simulink model "PILEncoder"  (R2021a)
settings: Solver=FixedStepAuto  StartTime=0.0  StopTime=41.24  FixedStep=0.001  RelTol=1e-3  EnableMultiTasking=on
values from neighbouring files (symbols this model uses):
  den_lpf_d = den_lpf20    [Mainframe_init.m]    (also in load_autopilot.m)
  Emulated_FCC_IO_Delay = 7    [Mainframe_init.m]
  Enable_Gyros = 0    [Mainframe_init.m]
  Enable_INS = 0    [Mainframe_init.m]
  num_lpf_d = num_lpf20    [Mainframe_init.m]    (also in load_autopilot.m)
undefined symbols (not defined in the file or in its folder): act_dmp, act_omega, Actuator, Aerodynamics, aMode, Autopilot, AUX, c_b_WGS, c_be, c_flat, c_grav, c_h_geop0, c_h_geope, c_pa0, c_pe, c_r0, c_rot, c_rsma, c_Tmp0, d_siB_0, d_siB_max, d_siB_min, dd_siB_max, dd_siB_min, dev, DiscIntNeverNeededParam, e_pa, e_Tmp, Earth, fin_maxrate, flag_I_act_switch, flag_I_aero_switch, flag_I_flat, flag_I_gravity_switch, flag_I_rot, Flight_Logic, hcr, HIL_Data, JMMM_0, JMMM_e, JSPB_e, lat_0, lon_0, Main, Mass_Props, mB_0, mM_0, mM_e, pBII_0, pMPB, pNPB, propellant_kg, prp_FBPB, prp_mdot, prp_T, pSPB, pwm_output0, pwm_output1, qEG_0, qIB_0 ... (+30)
libraries: simulink x42, simulink_extras x24, aerolibcommonsys x4, px4lib x2, custom_blocks x1, dspstat3 x1, pil_lib x1, aerolibtransform2 x1, dspnetwork x1, aerolibnav x1
(part 4 of 16)

== system PILEncoder/Non-linear Flight Dynamic Model/Subsystem1/Extract States/quaternion_to_euler_angles1 ==
  note: Um numerische Probleme zu
      | vermeiden, wird hier eine Saturiierung
      | benutzt.
  note: Outputs [size]:
      |
      | roll angle [1]
      | pitch angle [1]
      | yaw angle [1]
  note: Inputs [size]:
      |
      | quaternion [4]
  q : Inport  PortDimensions=4
  Add : Sum
  Add1 : Sum  Inputs=+--
  Add2 : Sum  Inputs=+-
  Add3 : Sum
  Add4 : Sum  Inputs=+--
  Complex to Real-Imag : ComplexToRealImag  Output=Real
  Constant : Constant  Value=0.5
  Constant1 : Constant  Value=0.5
  Demux : Demux
  Gain : Gain  Gain=2
  Product{,1..9} (10 alike) : Product
  Saturation : Saturate  UpperLimit=1  LowerLimit=-1
      settings: AttributesFormatString=|
      | %<UpperLimit>
      | %<LowerLimit>
  Trigonometric Function : Trigonometry  Operator=atan2
  Trigonometric Function1 : Trigonometry  Operator=asin
  Trigonometric Function2 : Trigonometry  Operator=atan2
  Vector Concatenate : Concatenate  NumInputs=3
  eulx : Outport  VectorParamsAs1DForOutWhenUnconnected=off
  wires:
  Vector Concatenate/1 -> Complex to Real-Imag/1
  Complex to Real-Imag/1 -> eulx/1
  Trigonometric Function2/1 -> Vector Concatenate/3
  Trigonometric Function1/1 -> Vector Concatenate/2
  Trigonometric Function/1 -> Vector Concatenate/1
  Add/1 -> Trigonometric Function/1
  Product1/1 -> Add/2
  Product/1 -> Add/1
  Product3/1 -> Add1/3
  Product2/1 -> Add1/2
  Product5/1 -> Add2/2
  Product4/1 -> Add2/1
  Product7/1 -> Add3/2
  Product6/1 -> Add3/1
  Add3/1 -> Trigonometric Function2/1
  Add4/1 -> Trigonometric Function2/2
  Add2/1 -> Gain/1
  Add1/1 -> Trigonometric Function/2
  q/1 -> Demux/1
  Demux/4 -> Product7/2, Product4/2, Product/2  "4"
  Demux/1 -> Product2/2, Product2/1, Product/1, Product6/1, Product5/1  "1"
  Demux/2 -> Product4/1, Product3/2, Product3/1, Product1/1, Product8/2, Product8/1, Product6/2  "2"
  Constant/1 -> Add1/1
  Product9/1 -> Add4/3
  Product8/1 -> Add4/2
  Constant1/1 -> Add4/1
  Demux/3 -> Product9/2, Product9/1, Product7/1, Product1/2, Product5/2  "3"
  Gain/1 -> Saturation/1
  Saturation/1 -> Trigonometric Function1/1

== system PILEncoder/Non-linear Flight Dynamic Model/Subsystem1/Fin Deflections/Degrees to Radians ==
  Degrees in : Inport
  Gain1 : Gain  Gain=pi/180  SaturateOnIntegerOverflow=on  OutDataTypeStr=Inherit: Same as input  ParamDataTypeStr=Inherit: Same as input
  Radians out : Outport  InitialOutput=0  VectorParamsAs1DForOutWhenUnconnected=off
  wires:
  Gain1/1 -> Radians out/1
  Degrees in/1 -> Gain1/1

== system PILEncoder/Non-linear Flight Dynamic Model/Subsystem1/Fin Deflections/Degrees to Radians1 ==
  Degrees in : Inport
  Gain1 : Gain  Gain=pi/180  SaturateOnIntegerOverflow=on  OutDataTypeStr=Inherit: Same as input  ParamDataTypeStr=Inherit: Same as input
  Radians out : Outport  InitialOutput=0  VectorParamsAs1DForOutWhenUnconnected=off
  wires:
  Gain1/1 -> Radians out/1
  Degrees in/1 -> Gain1/1

== system PILEncoder/Non-linear Flight Dynamic Model/Subsystem1/Fin Deflections/Degrees to Radians2 ==
  Degrees in : Inport
  Gain1 : Gain  Gain=pi/180  SaturateOnIntegerOverflow=on  OutDataTypeStr=Inherit: Same as input  ParamDataTypeStr=Inherit: Same as input
  Radians out : Outport  InitialOutput=0  VectorParamsAs1DForOutWhenUnconnected=off
  wires:
  Gain1/1 -> Radians out/1
  Degrees in/1 -> Gain1/1

== system PILEncoder/Non-linear Flight Dynamic Model/Subsystem1/Fin Deflections/control_allocation ==
  fin_cmd : Inport
  Constant7 : Constant  Value=Tr4r3
  Product : Product  Multiplication=Matrix(*)
  siB_cmd : Outport  VectorParamsAs1DForOutWhenUnconnected=off
  wires:
  Product/1 -> siB_cmd/1  "siB_cmd"
  fin_cmd/1 -> Product/2
  Constant7/1 -> Product/1

== system PILEncoder/Non-linear Flight Dynamic Model/Subsystem1/GRM_Airframe/aerodynamics ==
  str_flow : Inport
  fin : Inport  Port=2
  wab : Inport  Port=3
  env_glbl : Inport  Port=4
  Bus Selector : BusSelector  OutputSignals=qdynB,MaB,alB,beB,hBE,wBIB_star
  Bus Selector1 : BusSelector  OutputSignals=afinB
  Bus Selector2 : BusSelector  OutputSignals=pBPB
  aerodynamic_via_lookup : Subsystem
  logic_base_drag : Subsystem
  aero : Outport  VectorParamsAs1DForOutWhenUnconnected=off
  wires:
  str_flow/1 -> Bus Selector/1
  wab/1 -> Bus Selector2/1
  fin/1 -> Bus Selector1/1
  Bus Selector2/1 -> aerodynamic_via_lookup/1(pBPB)  "<pBPB>"
  Bus Selector/1 -> aerodynamic_via_lookup/2(qdynB)  "<qdynB>"
  Bus Selector/2 -> aerodynamic_via_lookup/3(MaB)  "<MaB>"
  Bus Selector/3 -> aerodynamic_via_lookup/4(alB)  "<alB>"
  Bus Selector/4 -> aerodynamic_via_lookup/5(beB)  "<beB>"
  Bus Selector/5 -> aerodynamic_via_lookup/6(hBE)  "<hBE>"
  Bus Selector1/1 -> aerodynamic_via_lookup/8(afinB)  "<afinB>"
  Bus Selector/6 -> aerodynamic_via_lookup/7(wBIB_star)  "<wBIB_star>"
  aerodynamic_via_lookup/1(aero_bus) -> aero/1
  env_glbl/1 -> logic_base_drag/1(env_glbl)
  logic_base_drag/1(flag_base_drag) -> aerodynamic_via_lookup/9(flag_I_prp)

== system PILEncoder/Non-linear Flight Dynamic Model/Subsystem1/GRM_Airframe/environment ==
  flight_dyn : Inport
  env_glbl : Inport  Port=2
  Bus Creator1 : BusCreator  Inputs=2
  Bus Creator2 : BusCreator  Inputs=2
  Bus Selector : BusSelector  OutputSignals=lon,lat,hBE
  Bus Selector1 : BusSelector  OutputSignals=atm_dyn_bus
  Saturation : Saturate  UpperLimit=inf  LowerLimit=eps
      settings: AttributesFormatString=|
      | %<UpperLimit>
      | %<LowerLimit>
  WGS84_Gravitation : Subsystem  mask{flg_omega_enabled=on}
      mask prompts: flg_omega_enabled "Zentripetalbeschleunigung mitberechnen"
      mask help:
      | Dieser Block berechnet die Gravitation für das idealisierte WGS84
      | Ellipsoid. Die Berechnung ist hierbei nach dem Technical Report
      | "Department of Defense World Geodetic System 1984", NIMA TR8350.2,
      | Third Edition, Amendment 1 vom 3 Januar 2000 implementiert.
      | Das Modell ist gültig für alle Höhen über dem WGS84 Referenzellipsoid, und
      | ist somit der reinen Taylorexpansion des Somigliana Modells überlegen
      | (siehe Kapitel 4.3 des WGS84 reports).
      |
      | ---------------------------------------------------------------------------
      | Longitude [rad]: Nach WGS84 definierte Geodätische Länge.  (lambda)
      | Lattitude [rad]: Nach WGS84 definierte Geodätische Breite. (phi)
      | Height [m]: Höhe über dem WGS84 Referenzellipsoid.
      mask init:
      | [ c_rsma, c_b_WGS, c_grav, c_rot] = init_WGS84_Gravitationsmodell();
  atmosphere_static_ISO_2533 : Subsystem
  convert_to_local_frame : Subsystem
  env : Outport  VectorParamsAs1DForOutWhenUnconnected=off
  wires:
  convert_to_local_frame/1(gBG) -> Bus Creator2/1
  flight_dyn/1 -> Bus Selector/1
  WGS84_Gravitation/1(gE) -> convert_to_local_frame/1(gE)
  Bus Selector/1 -> WGS84_Gravitation/1(lon)  "<lon>"
  Bus Selector/3 -> atmosphere_static_ISO_2533/1(hBE), Saturation/1  "<hBE>"
  Bus Creator2/1 -> env/1  "env_bus"
  Bus Selector/2 -> WGS84_Gravitation/2(lat)  "<lat>"
  Bus Creator1/1 -> Bus Creator2/2  "atm_bus"
  Saturation/1 -> WGS84_Gravitation/3(h)
  atmosphere_static_ISO_2533/1(atm_stat) -> Bus Creator1/1  "atm_stat_bus"
  env_glbl/1 -> Bus Selector1/1, atmosphere_static_ISO_2533/2(env_glbl)
  Bus Selector1/1 -> Bus Creator1/2  "<atm_dyn_bus>"

== system PILEncoder/Non-linear Flight Dynamic Model/Subsystem1/GRM_Airframe/fin_actuators ==
  cmd : Inport
  Bus Creator3 : BusCreator  Inputs=7
  Bus Selector : BusSelector  OutputSignals=siB_cmd
  Constant : Constant  Value=flag_I_act_switch
  Constant7 : Constant  Value=tRRR
  Demux : Demux
  Rudder : Subsystem  mask{siB_max=siB_max, siB_min=siB_min, d_siB_max=d_siB_max, d_siB_min=d_siB_min, dd_siB_max=dd_siB_max, dd_siB_min=dd_siB_min, omega=act_omega, dmp=act_dmp, unc_bl=unc_act_bl, unc_scale=unc_act_scale, unc_off=unc_act_off, siB_0=siB_0, d_siB_0=d_siB_0}
      mask prompts: siB_max "Obere Limitierung des Ruderstellwinkels in [rad]"; siB_min "Untere Limitierung des Ruderstellwinkels in [rad]"; d_siB_max "Obere Limitierung der Ruderstellwinkelgeschwindigkeit in [rad/s]"; d_siB_min "Untere Limitierung der Ruderstellwinkelgeschwindigkeit in [rad/s]"; dd_siB_max "Obere Limitierung der Ruderstellwinkelbeschleunigung in [rad/s^2]"; dd_siB_min "Untere Limitierung der Ruderstellwinkelbeschleunigung in [rad/s^2]"; omega "Eckfrequenz in [Hz]"; dmp "Dämpfung in [kg/s]"; unc_bl "Rückschlag des Aktuators (Backlash) in [rad]"; unc_scale "Skalenfehler in [-]"; unc_off "Versatz (Offset) in [rad]"; siB_0 "Startwert Ruderwinkel in [rad]"; d_siB_0 "Startwert Ruderwinkelgeschwindigkeiten in [rad/s]"
      mask DialogControl ParameterGroupVar Prompt: Limitierungen
      mask DialogControl Container3 Prompt: Dynamik
      mask DialogControl Container4 Prompt: Aktuatorfehler
      mask DialogControl Container5 Prompt: Startwerte
  Rudder1 : Subsystem  mask{siB_max=siB_max, siB_min=siB_min, d_siB_max=d_siB_max, d_siB_min=d_siB_min, dd_siB_max=dd_siB_max, dd_siB_min=dd_siB_min, omega=act_omega, dmp=act_dmp, unc_bl=unc_act_bl, unc_scale=unc_act_scale, unc_off=unc_act_off, siB_0=siB_0, d_siB_0=d_siB_0}
      mask prompts: siB_max "Obere Limitierung des Ruderstellwinkels in [rad]"; siB_min "Untere Limitierung des Ruderstellwinkels in [rad]"; d_siB_max "Obere Limitierung der Ruderstellwinkelgeschwindigkeit in [rad/s]"; d_siB_min "Untere Limitierung der Ruderstellwinkelgeschwindigkeit in [rad/s]"; dd_siB_max "Obere Limitierung der Ruderstellwinkelbeschleunigung in [rad/s^2]"; dd_siB_min "Untere Limitierung der Ruderstellwinkelbeschleunigung in [rad/s^2]"; omega "Eckfrequenz in [Hz]"; dmp "Dämpfung in [kg/s]"; unc_bl "Rückschlag des Aktuators (Backlash) in [rad]"; unc_scale "Skalenfehler in [-]"; unc_off "Versatz (Offset) in [rad]"; siB_0 "Startwert Ruderwinkel in [rad]"; d_siB_0 "Startwert Ruderwinkelgeschwindigkeiten in [rad/s]"
      mask DialogControl ParameterGroupVar Prompt: Limitierungen
      mask DialogControl Container3 Prompt: Dynamik
      mask DialogControl Container4 Prompt: Aktuatorfehler
      mask DialogControl Container5 Prompt: Startwerte
  Rudder2 : Subsystem  mask{siB_max=siB_max, siB_min=siB_min, d_siB_max=d_siB_max, d_siB_min=d_siB_min, dd_siB_max=dd_siB_max, dd_siB_min=dd_siB_min, omega=act_omega, dmp=act_dmp, unc_bl=unc_act_bl, unc_scale=unc_act_scale, unc_off=unc_act_off, siB_0=siB_0, d_siB_0=d_siB_0}
      mask prompts: siB_max "Obere Limitierung des Ruderstellwinkels in [rad]"; siB_min "Untere Limitierung des Ruderstellwinkels in [rad]"; d_siB_max "Obere Limitierung der Ruderstellwinkelgeschwindigkeit in [rad/s]"; d_siB_min "Untere Limitierung der Ruderstellwinkelgeschwindigkeit in [rad/s]"; dd_siB_max "Obere Limitierung der Ruderstellwinkelbeschleunigung in [rad/s^2]"; dd_siB_min "Untere Limitierung der Ruderstellwinkelbeschleunigung in [rad/s^2]"; omega "Eckfrequenz in [Hz]"; dmp "Dämpfung in [kg/s]"; unc_bl "Rückschlag des Aktuators (Backlash) in [rad]"; unc_scale "Skalenfehler in [-]"; unc_off "Versatz (Offset) in [rad]"; siB_0 "Startwert Ruderwinkel in [rad]"; d_siB_0 "Startwert Ruderwinkelgeschwindigkeiten in [rad/s]"
      mask DialogControl ParameterGroupVar Prompt: Limitierungen
      mask DialogControl Container3 Prompt: Dynamik
      mask DialogControl Container4 Prompt: Aktuatorfehler
      mask DialogControl Container5 Prompt: Startwerte
  Rudder3 : Subsystem  mask{siB_max=siB_max, siB_min=siB_min, d_siB_max=d_siB_max, d_siB_min=d_siB_min, dd_siB_max=dd_siB_max, dd_siB_min=dd_siB_min, omega=act_omega, dmp=act_dmp, unc_bl=unc_act_bl, unc_scale=unc_act_scale, unc_off=unc_act_off, siB_0=siB_0, d_siB_0=d_siB_0}
      mask prompts: siB_max "Obere Limitierung des Ruderstellwinkels in [rad]"; siB_min "Untere Limitierung des Ruderstellwinkels in [rad]"; d_siB_max "Obere Limitierung der Ruderstellwinkelgeschwindigkeit in [rad/s]"; d_siB_min "Untere Limitierung der Ruderstellwinkelgeschwindigkeit in [rad/s]"; dd_siB_max "Obere Limitierung der Ruderstellwinkelbeschleunigung in [rad/s^2]"; dd_siB_min "Untere Limitierung der Ruderstellwinkelbeschleunigung in [rad/s^2]"; omega "Eckfrequenz in [Hz]"; dmp "Dämpfung in [kg/s]"; unc_bl "Rückschlag des Aktuators (Backlash) in [rad]"; unc_scale "Skalenfehler in [-]"; unc_off "Versatz (Offset) in [rad]"; siB_0 "Startwert Ruderwinkel in [rad]"; d_siB_0 "Startwert Ruderwinkelgeschwindigkeiten in [rad/s]"
      mask DialogControl ParameterGroupVar Prompt: Limitierungen
      mask DialogControl Container3 Prompt: Dynamik
      mask DialogControl Container4 Prompt: Aktuatorfehler
      mask DialogControl Container5 Prompt: Startwerte
  Switch : Switch  Criteria=u2 > Threshold
  Vector Concatenate1 : Concatenate  NumInputs=4
  Vector Concatenate2 : Concatenate  NumInputs=4
  Vector Concatenate3 : Concatenate  NumInputs=4
  control_allocation : Subsystem
  fin : Outport  VectorParamsAs1DForOutWhenUnconnected=off
  wires:
  [d_siB3] -> Vector Concatenate2/3
  Demux/4 -> Rudder3/1(siB_c)
  Rudder2/2(d_siB) -> [d_siB3]
  Rudder3/1(siB) -> Vector Concatenate1/4
  Rudder1/2(d_siB) -> [d_siB2]
  Rudder2/1(siB) -> Vector Concatenate1/3
  [d_siB4] -> Vector Concatenate2/4
  [d_siB1] -> Vector Concatenate2/1
  Bus Selector/1 -> Switch/3, Demux/1  "<siB_cmd>"
  [d_siB2] -> Vector Concatenate2/2
  Constant7/1 -> Rudder1/2(tRRR), Rudder3/2(tRRR), Rudder2/2(tRRR), Rudder/2(tRRR)
  [dd_siB2] -> Vector Concatenate3/2
  Demux/3 -> Rudder2/1(siB_c)
  Rudder3/2(d_siB) -> [d_siB4]
  Demux/1 -> Rudder/1(siB_c)
  [dd_siB4] -> Vector Concatenate3/4
  [dd_siB3] -> Vector Concatenate3/3
  cmd/1 -> Bus Selector/1
  [dd_siB1] -> Vector Concatenate3/1
  Rudder1/1(siB) -> Vector Concatenate1/2
  Rudder1/3(dd_siB) -> [dd_siB2]
  Rudder3/3(dd_siB) -> [dd_siB4]
  Rudder/2(d_siB) -> [d_siB1]
  Rudder2/3(dd_siB) -> [dd_siB3]
  Demux/2 -> Rudder1/1(siB_c)
  Rudder/3(dd_siB) -> [dd_siB1]
  Rudder/1(siB) -> Vector Concatenate1/1
  Bus Creator3/1 -> fin/1  "fin_bus"
  Switch/1 -> Bus Creator3/1, control_allocation/1(siB)  "siB"
  Vector Concatenate2/1 -> control_allocation/2(d_siB), Bus Creator3/7  "d_siB"
  Vector Concatenate3/1 -> Bus Creator3/6, control_allocation/3(dd_siB)  "dd_siB"
  control_allocation/1(Tr3r4) -> Bus Creator3/2
  control_allocation/2(finB) -> Bus Creator3/3
  control_allocation/3(d_finB) -> Bus Creator3/4
  control_allocation/4(dd_finB) -> Bus Creator3/5
  Vector Concatenate1/1 -> Switch/1  "siB"
  Constant/1 -> Switch/2

== system PILEncoder/Non-linear Flight Dynamic Model/Subsystem1/GRM_Airframe/forces_moments ==
  aero : Inport
  motion_kin : Inport  Port=2
  grav : Inport  Port=3
  prp : Inport  Port=4
  Add : Sum  Inputs=+++
  Add1 : Sum
  Bus Creator : BusCreator  Inputs=2
  Bus Selector : BusSelector  OutputSignals=FBAB,MBAB
  Bus Selector1 : BusSelector  OutputSignals=TGB
  Bus Selector2 : BusSelector  OutputSignals=FBGG
  Bus Selector3 : BusSelector  OutputSignals=FBPB,MBPB
  Math Function : Math  Operator=transpose  SignedPower=on  SaturateOnIntegerOverflow=on
  Product : Product  Multiplication=Matrix(*)
  for_mom_bus : Outport  VectorParamsAs1DForOutWhenUnconnected=off
  wires:
  Bus Selector/1 -> Add/1  "<FBAB>"
  Bus Selector2/1 -> Product/2  "<FBGG>"
  Bus Selector1/1 -> Math Function/1  "<TGB>"
  Math Function/1 -> Product/1  "TBG"
  aero/1 -> Bus Selector/1
  Product/1 -> Add/2  "FBGB"
  prp/1 -> Bus Selector3/1
  motion_kin/1 -> Bus Selector1/1
  Add/1 -> Bus Creator/1  "FBTB"
  grav/1 -> Bus Selector2/1
  Add1/1 -> Bus Creator/2  "MBTB"
  Bus Selector/2 -> Add1/1  "<MBAB>"
  Bus Selector3/1 -> Add/3  "<FBPB>"
  Bus Creator/1 -> for_mom_bus/1  "for_mom_bus"
  Bus Selector3/2 -> Add1/2  "<MBPB>"

== system PILEncoder/Non-linear Flight Dynamic Model/Subsystem1/GRM_Airframe/gravity ==
  env : Inport
  wab : Inport  Port=2
  Bus Creator3 : BusCreator  Inputs=1
  Bus Selector : BusSelector  OutputSignals=gBG,atm_bus.atm_stat_bus.hBE
  Bus Selector1 : BusSelector  OutputSignals=mB
  Product : Product
  launch_rail : Subsystem
  grav : Outport  VectorParamsAs1DForOutWhenUnconnected=off
  wires:
  launch_rail/1(gBG) -> Product/1
  Bus Selector/2 -> launch_rail/2(hBE)  "<hBE>"
  Bus Selector/1 -> launch_rail/1(gBG_c)  "<gBG>"
  Product/1 -> Bus Creator3/1  "FBGG"
  Bus Creator3/1 -> grav/1  "grav_bus"
  wab/1 -> Bus Selector1/1
  Bus Selector1/1 -> Product/2  "<mB>"
  env/1 -> Bus Selector/1

== system PILEncoder/Non-linear Flight Dynamic Model/Subsystem1/GRM_Airframe/input ==
  siB_cmd : Inport
  Bus Creator2 : BusCreator  Inputs=1
  cmd_bus : Outport  VectorParamsAs1DForOutWhenUnconnected=off
  wires:
  siB_cmd/1 -> Bus Creator2/1
  Bus Creator2/1 -> cmd_bus/1  "cmd_bus"

== system PILEncoder/Non-linear Flight Dynamic Model/Subsystem1/GRM_Airframe/motion_kinematics ==
  flight_dyn : Inport
  Bus Creator : BusCreator  Inputs=7
  Bus Selector : BusSelector  OutputSignals=lat,lon,qIB
  calc_motion_kinematics : Subsystem
  motion_kin : Outport  VectorParamsAs1DForOutWhenUnconnected=off
  wires:
  flight_dyn/1 -> Bus Selector/1
  Bus Creator/1 -> motion_kin/1  "motion_kin_bus"
  Bus Selector/1 -> calc_motion_kinematics/1(lat)  "<lat>"
  Bus Selector/2 -> calc_motion_kinematics/2(lon)  "<lon>"
  Bus Selector/3 -> calc_motion_kinematics/3(qIB)  "<qIB>"
  calc_motion_kinematics/1(wIEE) -> Bus Creator/1
  calc_motion_kinematics/2(TIE) -> Bus Creator/2
  calc_motion_kinematics/3(TEB) -> Bus Creator/3
  calc_motion_kinematics/4(TGB) -> Bus Creator/4
  calc_motion_kinematics/5(TEG) -> Bus Creator/5
  calc_motion_kinematics/6(wEGG) -> Bus Creator/6
  calc_motion_kinematics/7(TIB) -> Bus Creator/7

== system PILEncoder/Non-linear Flight Dynamic Model/Subsystem1/GRM_Airframe/propulsion ==
  env_glbl : Inport
  wab : Inport  Port=2
  Bus Creator1 : BusCreator  Inputs=2
  prp_look_up : Subsystem
  prp_uncertainty : Subsystem
  prp : Outport  VectorParamsAs1DForOutWhenUnconnected=off
  wires:
  Bus Creator1/1 -> prp/1  "prp_bus"
  prp_look_up/1(FBPM) -> prp_uncertainty/1(FBPM)
  env_glbl/1 -> prp_look_up/1(env_glbl_bus)
  prp_uncertainty/2(MBPB) -> Bus Creator1/2
  prp_uncertainty/1(FBPB) -> Bus Creator1/1
  wab/1 -> prp_uncertainty/2(wab)

== system PILEncoder/Non-linear Flight Dynamic Model/Subsystem1/GRM_Airframe/rb_eom ==
  mot_kin : Inport
  for_mom : Inport  Port=2
  wab : Inport  Port=3
  Bus Creator : BusCreator  Inputs=16
  calc_bus_flight_dyn_bus_entries : Subsystem
  eom_6dof : Subsystem
  flight_dyn : Outport  VectorParamsAs1DForOutWhenUnconnected=off
  wires:
  mot_kin/1 -> calc_bus_flight_dyn_bus_entries/1(mot_kin)
  calc_bus_flight_dyn_bus_entries/1(aBIB) -> Bus Creator/1
  calc_bus_flight_dyn_bus_entries/2(lon) -> Bus Creator/2
  calc_bus_flight_dyn_bus_entries/3(lat) -> Bus Creator/3
  calc_bus_flight_dyn_bus_entries/4(hBE) -> Bus Creator/4
  calc_bus_flight_dyn_bus_entries/5(vBII) -> Bus Creator/5
  calc_bus_flight_dyn_bus_entries/6(qIB) -> Bus Creator/6
  calc_bus_flight_dyn_bus_entries/7(wBIB) -> Bus Creator/7
  calc_bus_flight_dyn_bus_entries/8(d_wBIB) -> Bus Creator/8
  calc_bus_flight_dyn_bus_entries/9(d_vBII) -> Bus Creator/9
  Bus Creator/1 -> flight_dyn/1  "flight_dyn_bus"
  for_mom/1 -> eom_6dof/1(for_mom)
  wab/1 -> eom_6dof/2(wab)
  eom_6dof/1(eom) -> calc_bus_flight_dyn_bus_entries/2(eom)
  calc_bus_flight_dyn_bus_entries/10(pBII) -> Bus Creator/10
  calc_bus_flight_dyn_bus_entries/11(euIB) -> Bus Creator/11
  calc_bus_flight_dyn_bus_entries/12(vBIB) -> Bus Creator/12
  calc_bus_flight_dyn_bus_entries/13(qGB) -> Bus Creator/13
  calc_bus_flight_dyn_bus_entries/14(euGB) -> Bus Creator/14
  calc_bus_flight_dyn_bus_entries/15(euBG) -> Bus Creator/15
  calc_bus_flight_dyn_bus_entries/16(pBLG) -> Bus Creator/16

== system PILEncoder/Non-linear Flight Dynamic Model/Subsystem1/GRM_Airframe/stream_flow ==
  flight_dyn : Inport
  motion_kin : Inport  Port=2
  env : Inport  Port=3
  Bus Selector1 : BusSelector  OutputSignals=atm_bus.atm_stat_bus.rho,atm_bus.atm_stat_bus.sos,atm_bus.atm_stat_bus.hBE
  Bus Selector2 : BusSelector  OutputSignals=vBII,pBII,wBIB
  Bus Selector3 : BusSelector  OutputSignals=TIB,wIEE,TIE
  calc_stream_flow : Subsystem
  str_flow : Outport  VectorParamsAs1DForOutWhenUnconnected=off
  wires:
  motion_kin/1 -> Bus Selector3/1
  flight_dyn/1 -> Bus Selector2/1
  env/1 -> Bus Selector1/1
  Bus Selector3/1 -> calc_stream_flow/1(TIB)  "<TIB>"
  Bus Selector3/2 -> calc_stream_flow/2(wIEE)  "<wIEE>"
  Bus Selector3/3 -> calc_stream_flow/3(TIE)  "<TIE>"
  Bus Selector2/1 -> calc_stream_flow/4(VBII)  "<vBII>"
  Bus Selector2/3 -> calc_stream_flow/6(wBIB)  "<wBIB>"
  Bus Selector1/1 -> calc_stream_flow/7(rho)  "<rho>"
  Bus Selector1/2 -> calc_stream_flow/8(sos)  "<sos>"
  Bus Selector1/3 -> calc_stream_flow/9(hBE)  "<hBE>"
  calc_stream_flow/1(str_flow) -> str_flow/1
  Bus Selector2/2 -> calc_stream_flow/5(pBII)  "<pBII>"

== system PILEncoder/Non-linear Flight Dynamic Model/Subsystem1/GRM_Airframe/weight_and_balance ==
  env_glb : Inport
  Bus Creator1 : BusCreator  Inputs=3
  Bus Selector2 : BusSelector  OutputSignals=T_sim_glbl,T_sim_lnch
  Subtract : Sum  Inputs=+-
  center_of_gravity : Subsystem
  mass : Subsystem
  mass_uncertainty : Subsystem
  moi : Subsystem
  wab : Outport  VectorParamsAs1DForOutWhenUnconnected=off
  wires:
  Bus Selector2/2 -> Subtract/2  "<T_sim_lnch>"
  Bus Selector2/1 -> Subtract/1  "<T_sim_glbl>"
  env_glb/1 -> Bus Selector2/1
  Bus Creator1/1 -> wab/1  "wab_bus"
  center_of_gravity/1(pBPB) -> moi/1(pBPB), Bus Creator1/2
  moi/1(JBBB) -> Bus Creator1/3
  mass/2(mM) -> moi/2(mM), center_of_gravity/2(mM)
  mass_uncertainty/1(mB) -> center_of_gravity/1(mB), Bus Creator1/1
  mass/1(mB_c) -> mass_uncertainty/1(mB_c)
  Subtract/1 -> mass/1(sim_time_launch)

== system PILEncoder/Flight Control Computer/FCC - Real or Emulated/Emulated FCC/P2R5/Emulated Pixhawk ==
  Serial In : Inport
  100 Hz : DiscretePulseGenerator  PulseType=Time based  Period=0.01  PulseWidth=50
  Autopilot : Subsystem
  Convert to Bus : Subsystem
  Convert to Vector : Subsystem
  IMU - Merge : Subsystem
  Inertial Navigation System : Subsystem
  Real Gyro : Subsystem
  Servo Commands : Subsystem
  Terminator : Terminator
  Zero : Constant  Value=0  OutDataTypeStr=Inherit: Inherit via back propagation
  Serial Out : Outport
  flight_mode_enum : Outport  Port=2
  tag scope: Heartbeat=global
  wires:
  [Heartbeat] -> Convert to Vector/2(Heartbeat)
  [INS_Data] -> Convert to Vector/3(INS Data)
  Serial In/1 -> Convert to Bus/1(Input)
  Convert to Vector/1(To HIL) -> Serial Out/1
  Convert to Bus/4(Missile States) -> Inertial Navigation System/2(Missile States)
  Convert to Bus/6(Virtual IMU Data) -> Real Gyro/1(HIL Gyro), IMU - Merge/1(HIL IMU)
  [INS_Data] -> Autopilot/3(INS Data)
  Real Gyro/1(Gyro Data) -> [Real_Gyro_Data]
  [Real_Gyro_Data] -> Convert to Vector/4(Real Gyro Data)
  [IMU_Data] -> Autopilot/2(IMU Data)
  Inertial Navigation System/1(INS Data) -> [INS_Data]
  Convert to Bus/3(Enable INS Flag) -> Inertial Navigation System/1(Enable INS Flag)
  Convert to Bus/5(Real Gyros Flag) -> Terminator/1
  Convert to Bus/2(Ext. Commands) -> [Ext_Cmd]
  Zero/1 -> Convert to Vector/5(Debug Port)
  IMU - Merge/1(IMU Data) -> [IMU_Data], Inertial Navigation System/3(IMU Data)
  Convert to Bus/1(Heartbeat) -> [Heartbeat]
  [Ext_Cmd] -> Autopilot/1(Cmd)
  Autopilot/1(Fin Deflections) -> Convert to Vector/1(Fin Deflections)
  Autopilot/2(flight_mode_enum) -> flight_mode_enum/1
  100 Hz/1 -> Autopilot/Trigger
  Autopilot/3(Fin Cmd) -> Servo Commands/1(Fin Cmd)
  Autopilot/4(Recovery) -> Servo Commands/2(Recovery)

== system PILEncoder/Flight Control Computer/FCC - Real or Emulated/Real FCC/P2R5/__InputSSForSFun__ ==
  Serial In : Inport
  __UniqueOutportName__1__ : Outport
  wires:
  Serial In/1 -> __UniqueOutportName__1__/1

== system PILEncoder/Flight Control Computer/FCC - Real or Emulated/Real FCC/P2R5/__OutputSSForSFun__ ==
  __UniqueInportName__1__ : Inport
  __UniqueInportName__2__ : Inport  Port=2
  Serial Out : Outport
  flight_mode_enum : Outport  Port=2
  wires:
  __UniqueInportName__2__/1 -> flight_mode_enum/1  "flight_mode_enum"
  __UniqueInportName__1__/1 -> Serial Out/1

== system PILEncoder/Flight Control Computer/FCC - Real or Emulated/Real FCC/PixBlock2/Emulated Pixhawk ==
  Serial In : Inport
  Trigger : TriggerPort  VariantControl=Variant  PortDimensions=1
  Autopilot : Subsystem
  Convert to Bus : Subsystem
  Convert to Vector : Subsystem
  Fin Allocation : Subsystem
  IMU - Merge : Subsystem
  Inertial Navigation System : Subsystem
  Real Gyro : Subsystem
  Servo Commands : Subsystem  Commented=on
  Terminator : Terminator
  Zero : Constant  Value=0  OutDataTypeStr=Inherit: Inherit via back propagation
  Serial Out : Outport
  tag scope: Heartbeat=global
  wires:
  [Heartbeat] -> Convert to Vector/2(Heartbeat)
  [INS_Data] -> Convert to Vector/3(INS Data)
  Serial In/1 -> Convert to Bus/1(Input)
  Convert to Vector/1(To HIL) -> Serial Out/1
  Convert to Bus/4(Missile States) -> Inertial Navigation System/2(Missile States)
  Convert to Bus/6(Virtual IMU Data) -> Real Gyro/1(HIL Gyro), IMU - Merge/1(HIL IMU)
  [INS_Data] -> Autopilot/3(INS Data)
  Real Gyro/1(Gyro Data) -> [Real_Gyro_Data]
  Fin Allocation/1(Fin Cmd) -> Servo Commands/1(Fin Cmd), Convert to Vector/1(Fin Deflections)
  Autopilot/1(Attitude_Commands) -> Fin Allocation/1(Attitude Cmd)  "ATT_Cmd"
  [Real_Gyro_Data] -> Convert to Vector/4(Real Gyro Data)
  [IMU_Data] -> Autopilot/2(IMU Data)
  Inertial Navigation System/1(INS Data) -> [INS_Data]
  Convert to Bus/3(Enable INS Flag) -> Inertial Navigation System/1(Enable INS Flag)
  Convert to Bus/5(Real Gyros Flag) -> Terminator/1
  Convert to Bus/2(Ext. Commands) -> [Ext_Cmd]
  Zero/1 -> Convert to Vector/5(Debug Port)
  IMU - Merge/1(IMU Data) -> [IMU_Data], Inertial Navigation System/3(IMU Data)
  Convert to Bus/1(Heartbeat) -> [Heartbeat]
  [Ext_Cmd] -> Autopilot/1(Cmd)

== system PILEncoder/Non-linear Flight Dynamic Model/Environment/atm_dynamic/trafo_around_z_axis/1_rot_mat ==
  wi1 : Inport
  1. Rotation x-Achse : Subsystem
  1. Rotation y-Achse : Subsystem
  1. Rotation z-Achse : Subsystem
  Constant : Constant  Value=rot_1
  Multiport Switch : MultiPortSwitch
  T12 : Outport  VectorParamsAs1DForOutWhenUnconnected=off
  wires:
  Constant/1 -> Multiport Switch/1
  1. Rotation x-Achse/1(1Rot_Matrix_x) -> Multiport Switch/2
  1. Rotation y-Achse/1(1Rot_Matrix_y) -> Multiport Switch/3
  1. Rotation z-Achse/1(1Rot_Matrix_z) -> Multiport Switch/4
  wi1/1 -> 1. Rotation x-Achse/1(alpha1), 1. Rotation z-Achse/1(alpha1), 1. Rotation y-Achse/1(alpha1)
  Multiport Switch/1 -> T12/1  "T12"

== system PILEncoder/Non-linear Flight Dynamic Model/Extract States/Assemble_States_Bus1/Three-axis Inertial Measurement Unit3/Acceleration Conversion ==
  acceleration : Inport  Unit=m/s^2
  Unit Conversion : UnitConversion
  inherit : Outport  VectorParamsAs1DForOutWhenUnconnected=off
  wires:
  acceleration/1 -> Unit Conversion/1
  Unit Conversion/1 -> inherit/1

== system PILEncoder/Non-linear Flight Dynamic Model/Extract States/Assemble_States_Bus1/Three-axis Inertial Measurement Unit3/Three-axis Accelerometer ==
  Ab : Inport  Unit=m/s^2  PortDimensions=3
  p q r : Inport  Port=2  Unit=rad/s
  pdot qdot rdot : Inport  Port=3  Unit=rad/s^2
  CG : Inport  Port=4  Unit=m  PortDimensions=3
  g : Inport  Port=5  Unit=m/s^2
  Disallow CGS : UnitConfiguration  UnitSystemsStr=English,SI,SI (extended)  AllowAllUnitSystems=off
  Dynamics : Subsystem
  Gain : Gain  Gain=[1 -1 1]  SaturateOnIntegerOverflow=on  OutDataTypeStr=Inherit: Same as input  ParamDataTypeStr=Inherit: Same as input
  Measurement bias : Constant  Value=a_bias
  Product : Product  Multiplication=Matrix(*)  SaturateOnIntegerOverflow=on  OutDataTypeStr=Inherit: Same as first input
  Random bias : aerolibcommonsys/Tunable White Noise  pwr=a_pow  Ts=0.1  seed=a_seeds
      settings: SourceProductBaseCode=AE
  Reshape1 : Reshape
  Saturation : Saturate  UpperLimit=a_sath  LowerLimit=a_satl
  Scale factors & Cross-coupling errors : Constant  Value=a_sf_cc
  Sum : Sum  Inputs=+-++  SaturateOnIntegerOverflow=on
  Sum1 : Sum  Inputs=|++  SaturateOnIntegerOverflow=on
  Sum4 : Sum  Inputs=++|  SaturateOnIntegerOverflow=on
  Sum7 : Sum  Inputs=|+-  SaturateOnIntegerOverflow=on
  Zero-Order Hold{,1..4} (5 alike) : Gain  SaturateOnIntegerOverflow=on  OutDataTypeStr=Inherit: Same as input  ParamDataTypeStr=Inherit: Same as input
  w x (w x d) : Subsystem
  wdot x d : Subsystem  mask(CrossProduct){aMode=aMode}
      mask help: shared_aeroblks:sharedaeroblkutil:blockCrossProductDesc
      mask init:
      | if aerosharedtest(gcb)
      |     aerosharedicon('shared');
      | else
      |     sharedautoicon('shared');
      | end
      mask Help: eval('if license(''test'',''Aerospace_Blockset'')aerosharedhelp(''threebythree_cross_product'');elseif license(''test'',''Powertrain_Blockset'')sharedautohelp(''threebythree_cross_product'');end')
      mask Display:
      | text(.5,.5,'Cross\nProduct\nC = AxB', ...
      | 	'HorizontalAlignment','Center',...
      | 	'VerticalAlignment','middle')
  wl_ins : Constant  Value=acc
  Ameas : Outport  Unit=m/s^2  PortDimensions=3  VectorParamsAs1DForOutWhenUnconnected=off
  wires:
  Zero-Order Hold4/1 -> Sum7/1
  Zero-Order Hold3/1 -> wdot x d/1(A)
  Zero-Order Hold/1 -> w x (w x d)/1("p q r ")
  Zero-Order Hold2/1 -> Sum/2
  Zero-Order Hold1/1 -> Sum/1
  g/1 -> Zero-Order Hold2/1
  Gain/1 -> wdot x d/2(B), w x (w x d)/2(distance)
  wl_ins/1 -> Sum7/2
  Sum7/1 -> Gain/1
  Dynamics/1("sp_f ") -> Sum1/1
  Sum4/1 -> Dynamics/1(sp_f)
  Sum1/1 -> Saturation/1
  w x (w x d)/1(w x ( w x d)) -> Sum/3
  Ab/1 -> Zero-Order Hold1/1
  Reshape1/1 -> Sum4/1
  Measurement bias/1 -> Sum4/2
  Product/1 -> Reshape1/1
  CG/1 -> Zero-Order Hold4/1
  pdot qdot rdot/1 -> Zero-Order Hold3/1
  p q r/1 -> Zero-Order Hold/1
  Sum/1 -> Product/2
  wdot x d/1(C) -> Sum/4
  Scale factors & Cross-coupling errors/1 -> Product/1
  Random bias/1 -> Sum1/2
  Saturation/1 -> Ameas/1

== system PILEncoder/Non-linear Flight Dynamic Model/Extract States/Assemble_States_Bus1/Three-axis Inertial Measurement Unit3/Three-axis Gyroscope ==
  p q r : Inport  Unit=rad/s  PortDimensions=3
  G's : Inport  Port=2  Unit=gn  PortDimensions=3
  Disallow CGS : UnitConfiguration  UnitSystemsStr=English,SI,SI (extended)  AllowAllUnitSystems=off
  Dynamics : Subsystem
  Measurement bias : Constant  Value=g_bias
  Product : Product  Multiplication=Matrix(*)  SaturateOnIntegerOverflow=on  OutDataTypeStr=Inherit: Same as first input
  Product1 : Product  SaturateOnIntegerOverflow=on  OutDataTypeStr=Inherit: Same as first input
  Random bias : aerolibcommonsys/Tunable White Noise  pwr=g_pow  Ts=0.1  seed=g_seeds
      settings: SourceProductBaseCode=AE
  Saturation : Saturate  UpperLimit=g_sath  LowerLimit=g_satl
  "Scale factors & Cross-coupling errors " : Constant  Value=g_sf_cc
  Sum1 : Sum  Inputs=|++  SaturateOnIntegerOverflow=on
  Sum4 : Sum  Inputs=+++  SaturateOnIntegerOverflow=on
  Zero-Order Hold : Gain  SaturateOnIntegerOverflow=on  OutDataTypeStr=Inherit: Same as input  ParamDataTypeStr=Inherit: Same as input
  Zero-Order Hold1 : Gain  SaturateOnIntegerOverflow=on  OutDataTypeStr=Inherit: Same as input  ParamDataTypeStr=Inherit: Same as input
  g-sensitive bias : Constant  Value=g_sen
  (p q r)_meas : Outport  Unit=rad/s  PortDimensions=3  VectorParamsAs1DForOutWhenUnconnected=off
  wires:
  Zero-Order Hold1/1 -> Product1/1
  Zero-Order Hold/1 -> Product/2
  Product1/1 -> Sum4/3
  Dynamics/1("p q r ") -> Sum1/1
  G's/1 -> Zero-Order Hold1/1
  Sum1/1 -> Saturation/1
  g-sensitive bias/1 -> Product1/2
  p q r/1 -> Zero-Order Hold/1
  Saturation/1 -> (p q r)_meas/1
  Random bias/1 -> Sum1/2
  "Scale factors & Cross-coupling errors "/1 -> Product/1
  Sum4/1 -> Dynamics/1(p q r)
  Product/1 -> Sum4/1
  Measurement bias/1 -> Sum4/2

== system PILEncoder/Non-linear Flight Dynamic Model/GRM_Airframe/aerodynamics/aerodynamic_via_lookup/calc_aero_coefficients ==
  dela_deg : Inport
  dele_deg : Inport  Port=2
  delr_deg : Inport  Port=3
  pBIB_star_rps : Inport  Port=4
  qBIB_star_rps : Inport  Port=5
  rBIB_star_rps : Inport  Port=6
  alB_deg : Inport  Port=7
  beB_deg : Inport  Port=8
  CLL_TLU : Subsystem
  CLM_TLU : Subsystem
  CLN_TLU : Subsystem
  CX_TLU : Subsystem
  CY_TLU : Subsystem
  CZ_TLU : Subsystem
  alB_deg D{1..5} (5 alike) : InportShadow  Port=7
  beB_deg D{1..5} (5 alike) : InportShadow  Port=8
  dela_deg D{1..6} (6 alike) : InportShadow
  dele_deg D{1..4} (4 alike) : InportShadow  Port=2
  delr_deg D{1..5} (5 alike) : InportShadow  Port=3
  Cx : Outport  VectorParamsAs1DForOutWhenUnconnected=off
  Cy : Outport  Port=2  VectorParamsAs1DForOutWhenUnconnected=off
  Cz : Outport  Port=3  VectorParamsAs1DForOutWhenUnconnected=off
  Cl : Outport  Port=4  VectorParamsAs1DForOutWhenUnconnected=off
  Cm : Outport  Port=5  VectorParamsAs1DForOutWhenUnconnected=off
  Cn : Outport  Port=6  VectorParamsAs1DForOutWhenUnconnected=off
  wires:
  CX_TLU/1(CX) -> Cx/1
  alB_deg/1 -> CX_TLU/1(alpha_deg)
  beB_deg/1 -> CX_TLU/2(beta_deg)
  dele_deg/1 -> CX_TLU/3(dele_deg)
  dela_deg/1 -> CX_TLU/4(dela_deg)
  CY_TLU/1(CY) -> Cy/1
  beB_deg D1/1 -> CY_TLU/2(beta_deg)
  alB_deg D1/1 -> CY_TLU/1(alpha_deg)
  delr_deg/1 -> CX_TLU/5(delr_deg)
  CZ_TLU/1(CZ) -> Cz/1
  CLL_TLU/1(CLL) -> Cl/1
  CLM_TLU/1(CLM) -> Cm/1
  CLN_TLU/1(CLN) -> Cn/1
  pBIB_star_rps/1 -> CLL_TLU/6(p_ND_rps)
  qBIB_star_rps/1 -> CLM_TLU/6(q_ND_rps)
  rBIB_star_rps/1 -> CLN_TLU/6(r_ND_rps)
  alB_deg D2/1 -> CZ_TLU/1(alpha_deg)
  beB_deg D2/1 -> CZ_TLU/2(beta_deg)
  dele_deg D1/1 -> CY_TLU/3(dele_deg)
  dela_deg D1/1 -> CY_TLU/4(dela_deg)
  delr_deg D1/1 -> CY_TLU/5(delr_deg)
  dele_deg D2/1 -> CZ_TLU/3(dele_deg)
  dela_deg D2/1 -> CZ_TLU/4(dela_deg)
  delr_deg D2/1 -> CZ_TLU/5(delr_deg)
  dela_deg D3/1 -> CLN_TLU/3(dele_deg)
  dela_deg D4/1 -> CLN_TLU/4(dela_deg)
  delr_deg D3/1 -> CLN_TLU/5(delr_deg)
  alB_deg D5/1 -> CLN_TLU/1(alpha_deg)
  alB_deg D4/1 -> CLM_TLU/1(alpha_deg)
  alB_deg D3/1 -> CLL_TLU/1(alpha_deg)
  beB_deg D3/1 -> CLL_TLU/2(beta_deg)
  beB_deg D4/1 -> CLM_TLU/2(beta_deg)
  beB_deg D5/1 -> CLN_TLU/2(beta_deg)
  dele_deg D3/1 -> CLL_TLU/3(dele_deg)
  dele_deg D4/1 -> CLM_TLU/3(dele_deg)
  dela_deg D5/1 -> CLL_TLU/4(dela_deg)
  dela_deg D6/1 -> CLM_TLU/4(dela_deg)
  delr_deg D4/1 -> CLL_TLU/5(delr_deg)
  delr_deg D5/1 -> CLM_TLU/5(delr_deg)

== system PILEncoder/Non-linear Flight Dynamic Model/GRM_Airframe/aerodynamics/aerodynamic_via_lookup/calc_aero_for_mom ==
  hBE : Inport
  pBPB : Inport  Port=2
  qdynB : Inport  Port=3
  Cx : Inport  Port=4
  Cy : Inport  Port=5
  Cz : Inport  Port=6
  Cl : Inport  Port=7
  Cm : Inport  Port=8
  Cn : Inport  Port=9
  Add : Sum
  Constant1 : Constant  Value=Aerodynamics.lref
      settings: AttributesFormatString=%<Value>
  Constant2 : Constant  Value=Aerodynamics.sref
      settings: AttributesFormatString=%<Value>
  Product : Product
  Product1 : Product  Inputs=3
  Product2 : Product
  Subtract : Sum  Inputs=+-
  Vector Concatenate1 : Concatenate  NumInputs=3
  Vector Concatenate2 : Concatenate  NumInputs=3
  create_pAPB : Subsystem
  cross_product : Subsystem
      mask help: cross product r3 = r1 x r2
      mask Help:
      | Name:
      | 
      |     cross_product
      | 
      | Description:
      | 
      |     This block implements the cross product r3 = r1 x r2.
      | 
      | Inputs  [size] [data type] [unit]:
      | 
      |     vector 1  [3] [double] [-]
      |     vector 2  [3] [double] [-]
      | 
      | Outputs  [size] [data type] [unit]:
      | 
      |     resulting vector  [3] [double] [-]
      mask Display: disp(' r3 = r1 x r2')
  launch_rail : Subsystem
  launch_rail1 : Subsystem
  FBAB : Outport  VectorParamsAs1DForOutWhenUnconnected=off
  MBAB : Outport  Port=2  VectorParamsAs1DForOutWhenUnconnected=off
  wires:
  Cy/1 -> Vector Concatenate2/2
  Cm/1 -> Vector Concatenate1/2
  Cz/1 -> Vector Concatenate2/3
  Cx/1 -> Vector Concatenate2/1
  Cl/1 -> Vector Concatenate1/1
  Cn/1 -> Vector Concatenate1/3
  qdynB/1 -> Product2/2
  Vector Concatenate1/1 -> Product1/2
  Vector Concatenate2/1 -> Product/1
  pBPB/1 -> Subtract/2
  Product/1 -> launch_rail/2(FBAB_c), cross_product/2(r2)  "FBAB"
  Product1/1 -> Add/2  "MBAB"
  Add/1 -> launch_rail1/2(MBAB_c)  "MBAB"
  Constant1/1 -> Product1/3
  Constant2/1 -> Product2/1
  Product2/1 -> Product1/1, Product/2
  cross_product/1(r1_x_r2) -> Add/1
  hBE/1 -> launch_rail1/1(hBE), launch_rail/1(hBE)
  launch_rail1/1(MBAB) -> MBAB/1
  launch_rail/1(FBAB) -> FBAB/1
  Subtract/1 -> cross_product/1(r1)  "pBAB"
  create_pAPB/1(pAPB) -> Subtract/1

== system PILEncoder/Non-linear Flight Dynamic Model/GRM_Airframe/environment/WGS84_Gravitation/WGS84_2_ECEF ==
  h : Inport
  lon : Inport  Port=2
  lat : Inport  Port=3
  Add1 : Sum  Inputs=+-
  Add2 : Sum
  Add3 : Sum
  Constant : Constant
  Divide : Product  Inputs=***
  Divide1 : Product  Inputs=***
  Divide2 : Product  Inputs=**
  Divide3 : Product  Inputs=**
  Divide4 : Product  Inputs=**
  Mux : Mux  Inputs=3
  Trigonometric Function : Trigonometry
  Trigonometric Function1 : Trigonometry  Operator=cos
  Trigonometric Function2 : Trigonometry
  Trigonometric Function3 : Trigonometry  Operator=cos
  "WGS84 Transformation Parameter " : Subsystem
  pE : Outport  VectorParamsAs1DForOutWhenUnconnected=off
  wires:
  Divide1/1 -> Mux/2  "y_ECEF"
  Add2/1 -> Divide4/1
  Divide/1 -> Mux/1  "x_ECEF"
  lat/1 -> "WGS84 Transformation Parameter "/1(phi), Trigonometric Function3/1, Trigonometric Function2/1
  Divide2/1 -> Add1/2
  Divide3/1 -> Add2/2  "N(1-e^2)"
  Constant/1 -> Add1/1
  Add1/1 -> Divide3/2
  Divide4/1 -> Mux/3  "z_ECEF"
  "WGS84 Transformation Parameter "/1(N) -> Add3/2, Divide3/1
  "WGS84 Transformation Parameter "/2(e) -> Divide2/2, Divide2/1
  h/1 -> Add2/1, Add3/1
  Trigonometric Function1/1 -> Divide/2  "cos(lambda)"
  Trigonometric Function3/1 -> Divide1/3, Divide/3  "cos(phi)"
  Mux/1 -> pE/1  "pE"
  lon/1 -> Trigonometric Function1/1, Trigonometric Function/1
  Add3/1 -> Divide1/1, Divide/1
  Trigonometric Function2/1 -> Divide4/2  "sin(phi)"
  Trigonometric Function/1 -> Divide1/2  "sin(lambda)"

== system PILEncoder/Non-linear Flight Dynamic Model/GRM_Airframe/environment/atmosphere_static_ISO_2533/density ==
  Tmp : Inport
  pa : Inport  Port=2
  Divide : Product  Inputs=/*/
  specific_gas_constant : Constant  Value=sgc
  rho : Outport  VectorParamsAs1DForOutWhenUnconnected=off
  wires:
  Tmp/1 -> Divide/1
  Divide/1 -> rho/1  "rho"
  pa/1 -> Divide/2
  specific_gas_constant/1 -> Divide/3

== system PILEncoder/Non-linear Flight Dynamic Model/GRM_Airframe/environment/atmosphere_static_ISO_2533/geopot_height ==
  hBE : Inport
  Add : Sum
  Divide : Product  Inputs=*/*
  mean_earth_radius : Constant  Value=mean_earth_radius
  h_geop : Outport  VectorParamsAs1DForOutWhenUnconnected=off
  wires:
  mean_earth_radius/1 -> Divide/3, Add/2
  Divide/1 -> h_geop/1  "h_geop"
  hBE/1 -> Add/1, Divide/1
  Add/1 -> Divide/2

== system PILEncoder/Non-linear Flight Dynamic Model/GRM_Airframe/environment/atmosphere_static_ISO_2533/speed_of_sound ==
  Tmp : Inport
  Product : Product  Inputs=3
  Sqrt : Sqrt  SaturateOnIntegerOverflow=on
  heat_capacity_ratio : Constant  Value=hcr
  specific_gas_constant : Constant  Value=sgc
  sos : Outport  VectorParamsAs1DForOutWhenUnconnected=off
  wires:
  Sqrt/1 -> sos/1  "sos"
  Tmp/1 -> Product/3
  Product/1 -> Sqrt/1
  heat_capacity_ratio/1 -> Product/2
  specific_gas_constant/1 -> Product/1

== system PILEncoder/Non-linear Flight Dynamic Model/GRM_Airframe/environment/atmosphere_static_ISO_2533/tmp_and_pressure_ISO_2533 ==
  h_geop : Inport
  e_Tmp : Inport  Port=2
  e_pa : Inport  Port=3
  Subtract1 : Sum
  Subtract2 : Sum
  Tmp_norm_msl : Constant  Value=c_Tmp0
  geopotential_height_ref : Constant  Value=c_h_geop0
  pa_norm_msl : Constant  Value=c_pa0
  static_Temperature : Subsystem
  static_pressure : Subsystem
  Tmp : Outport  VectorParamsAs1DForOutWhenUnconnected=off
  pa : Outport  Port=2  VectorParamsAs1DForOutWhenUnconnected=off
  wires:
  h_geop/1 -> static_pressure/2(h_geop), static_Temperature/2(h_geop)
  Subtract2/1 -> static_pressure/4(pa_ref)  "pa_ref"
  pa_norm_msl/1 -> Subtract2/2
  Subtract1/1 -> static_pressure/3(Tmp_ref), static_Temperature/1(Tmp_ref)  "Tmp_ref"
  static_pressure/1(pa) -> pa/1
  e_pa/1 -> Subtract2/1
  static_Temperature/1(Tmp) -> Tmp/1
  e_Tmp/1 -> Subtract1/1
  geopotential_height_ref/1 -> static_pressure/1(h_geop_ref), static_Temperature/3(h_geop_ref)  "h_geop_ref"
  Tmp_norm_msl/1 -> Subtract1/2

== system PILEncoder/Non-linear Flight Dynamic Model/GRM_Airframe/gravity/launch_rail/initial_altitude ==
  Constant : Constant  Value=pBII_0
  Constant2 : Constant  Value=flag_I_flat
  Demux : Demux  Outputs=3
  Gain : Gain  Gain=-1
  Switch1 : Switch  Criteria=u2 > Threshold
  Terminator{,1..3} (4 alike) : Terminator
  trafo_E_to_geodetic : Subsystem  mask(Transformation der ECEF Position in geodätische Größen){}
      mask help: Dieser Block transformiert die Position im ECEF KOS in die geodätische Länge, Breite und Höhe
      mask init:
      | [c_mue, c_rsma, c_flat] = init_transformations_earth;
      mask Help:
      | Name:
      | 
      |     trafo_E_to_geodetic
      | 
      | Beschreibung:
      | 
      |     Dieser Block transformiert die Position im ECEF KOS in die geodätische
      |     Länge, Breite und Höhe.
      | 
      | Inputs   [size]  [data type] [unit]:
      | 
      |     pBEE    [3] [double] [m]
      | 
      | Outputs  [size]  [data type] [unit]:
      | 
      |     long  [1] [double] [rad]
      |     lat   [1] [double] [rad]
      |     alt   [1] [double] [m]
      | 
      | Parameter
      | 
      |    c_rsma
      |    c_flat
  hBE_0 : Outport  VectorParamsAs1DForOutWhenUnconnected=off
  wires:
  Constant2/1 -> Switch1/2
  trafo_E_to_geodetic/3(alt) -> Switch1/3  "hBE_0"
  Demux/2 -> Terminator3/1
  Demux/3 -> Gain/1
  Gain/1 -> Switch1/1
  Demux/1 -> Terminator2/1
  trafo_E_to_geodetic/2(lat) -> Terminator1/1
  Constant/1 -> Demux/1, trafo_E_to_geodetic/1(pBEE)
  trafo_E_to_geodetic/1(lon) -> Terminator/1
  Switch1/1 -> hBE_0/1  "hBE_0"

== system PILEncoder/Non-linear Flight Dynamic Model/GRM_Airframe/motion_kinematics/calc_motion_kinematics/calc_transformation_matrix ==
  qIE : Inport
  qEG : Inport  Port=2
  qIB : Inport  Port=3
  T12_from_q1 : Subsystem
      mask help: Transforms a quaternion into a Direction Cosine Matrix
      mask Help:
      | Name:
      | 
      |     T12_from_q12
      | 
      | Description:
      | 
      |     This block implements the transformation of a quaternion into the
      |     corresponding direction cosine matrix DCM.
      | 
      | Inputs  [size] [data type] [unit]:
      | 
      |     quaternion q12 [4] [double] [-]
      | 
      | Outputs  [size] [data type] [unit]:
      | 
      |     direction cosine matrix T12  [3x3] [double] [-]
      mask Display:
      | %port_label('input', 1, 'q12')
      | %port_label('output', 1, 'T12')
      | disp('q \rightarrow DCM','texmode','on')
  T12_from_q12 : Subsystem
      mask help: Transforms a quaternion into a Direction Cosine Matrix
      mask Help:
      | Name:
      | 
      |     T12_from_q12
      | 
      | Description:
      | 
      |     This block implements the transformation of a quaternion into the
      |     corresponding direction cosine matrix DCM.
      | 
      | Inputs  [size] [data type] [unit]:
      | 
      |     quaternion q12 [4] [double] [-]
      | 
      | Outputs  [size] [data type] [unit]:
      | 
      |     direction cosine matrix T12  [3x3] [double] [-]
      mask Display:
      | %port_label('input', 1, 'q12')
      | %port_label('output', 1, 'T12')
      | disp('q \rightarrow DCM','texmode','on')
  T12_from_q2 : Subsystem
      mask help: Transforms a quaternion into a Direction Cosine Matrix
      mask Help:
      | Name:
      | 
      |     T12_from_q12
      | 
      | Description:
      | 
      |     This block implements the transformation of a quaternion into the
      |     corresponding direction cosine matrix DCM.
      | 
      | Inputs  [size] [data type] [unit]:
      | 
      |     quaternion q12 [4] [double] [-]
      | 
      | Outputs  [size] [data type] [unit]:
      | 
      |     direction cosine matrix T12  [3x3] [double] [-]
      mask Display:
      | %port_label('input', 1, 'q12')
      | %port_label('output', 1, 'T12')
      | disp('q \rightarrow DCM','texmode','on')
  conjugate_quaternion : Subsystem
      mask help: conjugate a quaternion
      mask Help:
      | Name:
      | 
      |     conjugate_quaternion
      | 
      | Description:
      | 
      |     computes the conjugate quaternion
      | 
      | Inputs  [size] [data type] [unit]:
      | 
      |     quaternion q_2_1  [4] [double] [-]
      | 
      | Outputs  [size] [data type] [unit]:
      | 
      |     conjugated quaternion q_1_2  [4] [double] [-]
      mask Display: disp (' conj(q)')
  q31_from_q32_mul_q1 : Subsystem
      mask help: multiply two quaternions
      mask Help:
      | Name:
      | 
      |     q31_from_q32_mul_q21
      | 
      | Description:
      | 
      |     This block implements the multiplication of two quaternions according
      |     to q31=q32*q21.
      | 
      | Inputs  [size] [data type] [unit]:
      | 
      |     attitude quaternion q32  [4] [double] [-]
      |     attitude quaternion q21  [4] [double] [-]
      | 
      | Outputs  [size] [data type] [unit]:
      | 
      |     attitude quaternion q31  [4] [double] [-]
      mask Display:
      | port_label('input', 1, 'q32')
      | port_label('input', 2, 'q21')
      | port_label('output', 1, 'q31')
      | disp('q_{31} = q_{32} {\bf\cdot} q_{21}','texmode','on')
  q31_from_q32_mul_q2 : Subsystem
      mask help: multiply two quaternions
      mask Help:
      | Name:
      | 
      |     q31_from_q32_mul_q21
      | 
      | Description:
      | 
      |     This block implements the multiplication of two quaternions according
      |     to q31=q32*q21.
      | 
      | Inputs  [size] [data type] [unit]:
      | 
      |     attitude quaternion q32  [4] [double] [-]
      |     attitude quaternion q21  [4] [double] [-]
      | 
      | Outputs  [size] [data type] [unit]:
      | 
      |     attitude quaternion q31  [4] [double] [-]
      mask Display:
      | port_label('input', 1, 'q32')
      | port_label('input', 2, 'q21')
      | port_label('output', 1, 'q31')
      | disp('q_{31} = q_{32} {\bf\cdot} q_{21}','texmode','on')
  q31_from_q32_mul_q21 : Subsystem
      mask help: multiply two quaternions
      mask Help:
      | Name:
      | 
      |     q31_from_q32_mul_q21
      | 
      | Description:
      | 
      |     This block implements the multiplication of two quaternions according
      |     to q31=q32*q21.
      | 
      | Inputs  [size] [data type] [unit]:
      | 
      |     attitude quaternion q32  [4] [double] [-]
      |     attitude quaternion q21  [4] [double] [-]
      | 
      | Outputs  [size] [data type] [unit]:
      | 
      |     attitude quaternion q31  [4] [double] [-]
      mask Display:
      | port_label('input', 1, 'q32')
      | port_label('input', 2, 'q21')
      | port_label('output', 1, 'q31')
      | disp('q_{31} = q_{32} {\bf\cdot} q_{21}','texmode','on')
  TEB : Outport  VectorParamsAs1DForOutWhenUnconnected=off
  TGB : Outport  Port=2  VectorParamsAs1DForOutWhenUnconnected=off
  TIB : Outport  Port=3  VectorParamsAs1DForOutWhenUnconnected=off
  wires:
  T12_from_q2/1(T12) -> TGB/1  "TGB"
  q31_from_q32_mul_q21/1(q31) -> conjugate_quaternion/1(q)  "qIG"
  qIB/1 -> q31_from_q32_mul_q1/2(q21), T12_from_q12/1(q12)
  q31_from_q32_mul_q1/1(q31) -> T12_from_q2/1(q12), q31_from_q32_mul_q2/2(q21)  "qGB"
  qEG/1 -> q31_from_q32_mul_q21/2(q21), q31_from_q32_mul_q2/1(q32)
  T12_from_q1/1(T12) -> TEB/1  "TEB"
  conjugate_quaternion/1(q_conj) -> q31_from_q32_mul_q1/1(q32)  "qGI"
  qIE/1 -> q31_from_q32_mul_q21/1(q32)
  q31_from_q32_mul_q2/1(q31) -> T12_from_q1/1(q12)  "qEB"
  T12_from_q12/1(T12) -> TIB/1  "TIB"
